simulink library "Spring_LeftRight_AsymmetricNonlinear"  (R2026a)
settings: Solver=VariableStepAuto
libraries: fl_lib x2, Spring_Nonlinear x2
Description:
  | Component of Simscape Vehicle Templates Library
  | 
  | Copyright 2018-2024 The MathWorks, Inc.
settings Model: Creator=smiller  LastModifiedBy=smiller

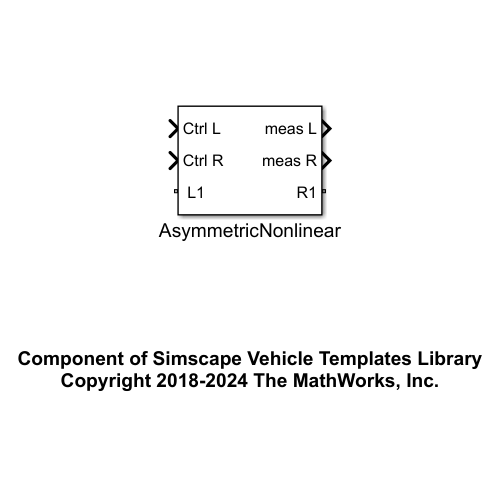
[thumbnail: Simulink's stored preview of the top-level diagram]
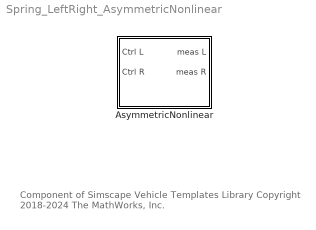
== system Spring_LeftRight_AsymmetricNonlinear ==
  note: Component of Simscape Vehicle Templates Library
      | Copyright 2018-2024 The MathWorks, Inc.
  AsymmetricNonlinear : Subsystem  VariantControl=Linear  mask(Asymmetric Nonlinear Springs){}
      mask help: Springs with independent hardpoint parameterization for left and right sides. For spring connections in suspensions that may be asymmetric at design position, such as panhard rod suspensions.

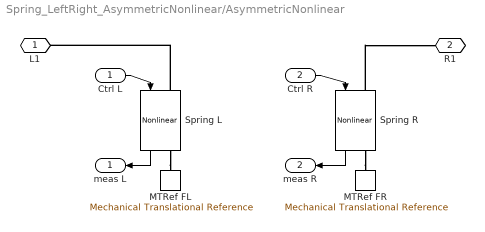
== system Spring_LeftRight_AsymmetricNonlinear/AsymmetricNonlinear ==
  Ctrl L : Inport
  Ctrl R : Inport  Port=2
  MTRef FL : fl_lib/Mechanical/Translational Elements/Mechanical Translational Reference
  MTRef FR : fl_lib/Mechanical/Translational Elements/Mechanical Translational Reference
  Spring L : Spring_Nonlinear/Nonlinear  VariantControl=Nonlinear  spr_frc0=Spring.fPreloadL.Value  deformation_vector=Spring.xSpringL.Value  force_vector=Spring.fSpringL.Value  spr_hp_top=Spring.sTopL.Value  spr_hp_bot=Spring.sBottomL.Value
  Spring R : Spring_Nonlinear/Nonlinear  VariantControl=Nonlinear  spr_frc0=Spring.fPreloadR.Value  deformation_vector=Spring.xSpringR.Value  force_vector=Spring.fSpringR.Value  spr_hp_top=Spring.sTopR.Value  spr_hp_bot=Spring.sBottomR.Value
  " L1" : PMIOPort  Side=Left
  R1 : PMIOPort  Port=2  Side=Right
  meas L : Outport  VectorParamsAs1DForOutWhenUnconnected=off
  meas R : Outport  Port=2  VectorParamsAs1DForOutWhenUnconnected=off
  wires:
  Ctrl L/1 -> Spring L/1
  Spring L/1 -> meas L/1
  Spring R/1 -> meas R/1
  Ctrl R/1 -> Spring R/1
  connections:
  Spring L/RConn1 -- MTRef FL/LConn1
  Spring R/RConn1 -- MTRef FR/LConn1
  Spring L/LConn1 -- " L1"/RConn1
  Spring R/LConn1 -- R1/RConn1
